simulink model "sf_tlat"  (Simulink 7.6)
settings: Solver=ode45  StartTime=0.0  StopTime=100  RelTol=1e-3
settings Model: Creator=The MathWorks Inc.  CovMetricSettings=dcmtr  ExtModeAutoUpdateStatusClock=off
settings OptimizationCC: BooleanDataType=off  InlineInvariantSignals=on  InitFltsAndDblsToZero=on  EfficientMapNaN2IntZero=off
settings DebuggingCC: SaveWithParameterizedLinksMsg=none  SignalResolutionControl=TryResolveAllWithWarning  SolverPrmCheckMsg=none  MultiTaskDSMMsg=warning  MultiTaskCondExecSysMsg=none  StrictBusMsg=None
settings HardwareCC: TargetUnknown=on
settings SFSimCC: SimParseCustomCode=off
settings RTWCC: IncludeERTFirstTime=on
settings GRTTargetCC: TargetFcnLib=ansi_tfl_tmw.mat

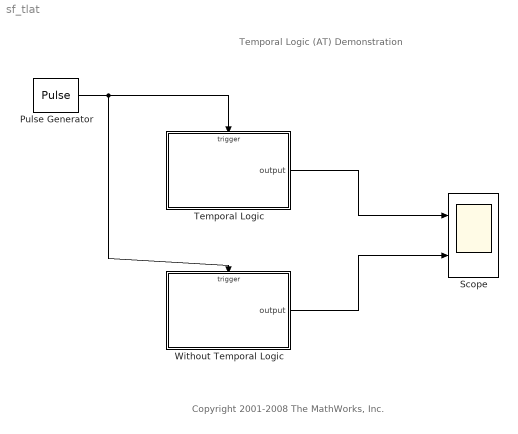
== system sf_tlat ==
  note: Temporal Logic (AT) Demonstration
  note: Copyright 2001-2008 The MathWorks, Inc.
  Pulse Generator : DiscretePulseGenerator  PulseType=Time based  Period=1  PulseWidth=50
  Scope : Scope  NumInputPorts=2
      settings: TimeRange=100  YMin=-1.5~-1.5  YMax=1.5~1.5
  Temporal Logic : Stateflow chart  TreatAsAtomicUnit=on
  Without Temporal Logic : Stateflow chart  TreatAsAtomicUnit=on
  wires:
  Pulse Generator/1 -> Temporal Logic/Trigger, Without Temporal Logic/Trigger
  Temporal Logic/1(output) -> Scope/1
  Without Temporal Logic/1(output) -> Scope/2

== stateflow chart Temporal Logic ==
  state State
    a=5;
    on at(a,event):output=1;
    on at(2*a,event):output=0;
  (default) -> State
  State -> (junction 4) : at(6*a,event)
  (junction 4) -> State : {output=-1;}
  data: output output double; a local double
  events: event input RISING_EDGE_EVENT

== stateflow chart Without Temporal Logic ==
  state A
    en: count = 1;
    A -> A [order 1] : {count++;a=count;}
  state B
    en:count=a+1;
    B -> B [order 1] : {count++;}
  state C
    en:count=2*a+1;
    C -> C [order 1] : {count++;}
  (default) -> A
  A -> B [order 1] : [count==5]{output=1;}
  B -> C [order 1] : [count==2*a]{output=0;}
  C -> A [order 1] : [count==6*a]{output=-1;}
  data: count local double; output output double; a local double
  events: control input RISING_EDGE_EVENT
